simulink model "EngPrt_PrtLimMech1"  (R2016b)
settings: configuration reference "CodeGenConfigSet" (kept outside this file)
values from neighbouring files (symbols this model uses):
  EngPrt_facEngSPOffset_CUR = Calibration.Parameter    [init_EngPrt_PrtLimMech.m]    (also in init_EngPrt_PrtLimMech_SIL.m = Simulink.Parameter)
  EngPrt_facEngSPOffset_CURX = Calibration.Parameter    [init_EngPrt_PrtLimMech.m]    (also in init_EngPrt_PrtLimMech_SIL.m = Simulink.Parameter)
  EngPrt_facTrqLimCor_MAP = Calibration.Parameter    [init_EngPrt_PrtLimMech.m]    (also in init_EngPrt_PrtLimMech_SIL.m = Simulink.Parameter)
  EngPrt_facTrqLimCor_MAPX = Calibration.Parameter    [init_EngPrt_PrtLimMech.m]    (also in init_EngPrt_PrtLimMech_SIL.m = Simulink.Parameter)
  EngPrt_facTrqLimCor_MAPY = Calibration.Parameter    [init_EngPrt_PrtLimMech.m]    (also in init_EngPrt_PrtLimMech_SIL.m = Simulink.Parameter)
  EngPrt_nEngSplimOffset_C = Calibration.Parameter    [init_EngPrt_PrtLimMech.m]    (also in init_EngPrt_PrtLimMech_SIL.m = Simulink.Parameter)
  EngPrt_nEngSplimRmpSlopeNeg_C = Calibration.Parameter    [init_EngPrt_PrtLimMech.m]    (also in init_EngPrt_PrtLimMech_SIL.m = Simulink.Parameter)
  EngPrt_nEngSplimRmpSlopePos_C = Calibration.Parameter    [init_EngPrt_PrtLimMech.m]    (also in init_EngPrt_PrtLimMech_SIL.m = Simulink.Parameter)
  EngPrt_numTrqLim_C = Calibration.Parameter    [init_EngPrt_PrtLimMech.m]    (also in init_EngPrt_PrtLimMech_SIL.m = Simulink.Parameter)
  EngPrt_qLim_CUR = Calibration.Parameter    [init_EngPrt_PrtLimMech.m]    (also in init_EngPrt_PrtLimMech_SIL.m = Simulink.Parameter)
  EngPrt_qLim_CURX = Calibration.Parameter    [init_EngPrt_PrtLimMech.m]    (also in init_EngPrt_PrtLimMech_SIL.m = Simulink.Parameter)
  EngPrt_RmpLimNErrNeg_C = Calibration.Parameter    [init_EngPrt_PrtLimMech.m]    (also in init_EngPrt_PrtLimMech_SIL.m = Simulink.Parameter)
  EngPrt_RmpLimNErrPos_C = Calibration.Parameter    [init_EngPrt_PrtLimMech.m]    (also in init_EngPrt_PrtLimMech_SIL.m = Simulink.Parameter)
  EngPrt_swtLimCorType_C = Calibration.Parameter    [init_EngPrt_PrtLimMech.m]    (also in init_EngPrt_PrtLimMech_SIL.m = Simulink.Parameter)
  EngPrt_swtTrq_C = Calibration.Parameter    [init_EngPrt_PrtLimMech.m]    (also in init_EngPrt_PrtLimMech_SIL.m = Simulink.Parameter)
  EngPrt_trqLim_CUR = Calibration.Parameter    [init_EngPrt_PrtLimMech.m]    (also in init_EngPrt_PrtLimMech_SIL.m = Simulink.Parameter)
  EngPrt_trqLim_CURX = Calibration.Parameter    [init_EngPrt_PrtLimMech.m]    (also in init_EngPrt_PrtLimMech_SIL.m = Simulink.Parameter)
  EngPrt_trqLimAPSCor_MAP = Calibration.Parameter    [init_EngPrt_PrtLimMech.m]    (also in init_EngPrt_PrtLimMech_SIL.m = Simulink.Parameter)
  EngPrt_trqLimAPSCor_MAPX = Calibration.Parameter    [init_EngPrt_PrtLimMech.m]    (also in init_EngPrt_PrtLimMech_SIL.m = Simulink.Parameter)
  EngPrt_trqLimAPSCor_MAPY = Calibration.Parameter    [init_EngPrt_PrtLimMech.m]    (also in init_EngPrt_PrtLimMech_SIL.m = Simulink.Parameter)
  EngPrt_trqLimEngTempCor_MAP = Calibration.Parameter    [init_EngPrt_PrtLimMech.m]    (also in init_EngPrt_PrtLimMech_SIL.m = Simulink.Parameter)
  EngPrt_trqLimEngTempCor_MAPX = Calibration.Parameter    [init_EngPrt_PrtLimMech.m]    (also in init_EngPrt_PrtLimMech_SIL.m = Simulink.Parameter)
  EngPrt_trqLimEngTempCor_MAPY = Calibration.Parameter    [init_EngPrt_PrtLimMech.m]    (also in init_EngPrt_PrtLimMech_SIL.m = Simulink.Parameter)
  EngPrt_trqNLim_CUR = Calibration.Parameter    [init_EngPrt_PrtLimMech.m]    (also in init_EngPrt_PrtLimMech_SIL.m = Simulink.Parameter)
  EngPrt_trqNLim_CURX = Calibration.Parameter    [init_EngPrt_PrtLimMech.m]    (also in init_EngPrt_PrtLimMech_SIL.m = Simulink.Parameter)
  EngPrt_trqNLimSpr_CUR = Calibration.Parameter    [init_EngPrt_PrtLimMech.m]    (also in init_EngPrt_PrtLimMech_SIL.m = Simulink.Parameter)
  EngPrt_trqNLimSpr_CURX = Calibration.Parameter    [init_EngPrt_PrtLimMech.m]    (also in init_EngPrt_PrtLimMech_SIL.m = Simulink.Parameter)
undefined symbols (not defined in the file or in its folder): EngPrt_PrtLimMech_DT, Switch_conv
libraries: CXLib x8
settings Model: Creator=Administrator  LastModifiedBy=xuxingpei
settings ConfigSetRef: SourceLocation=Base Workspace

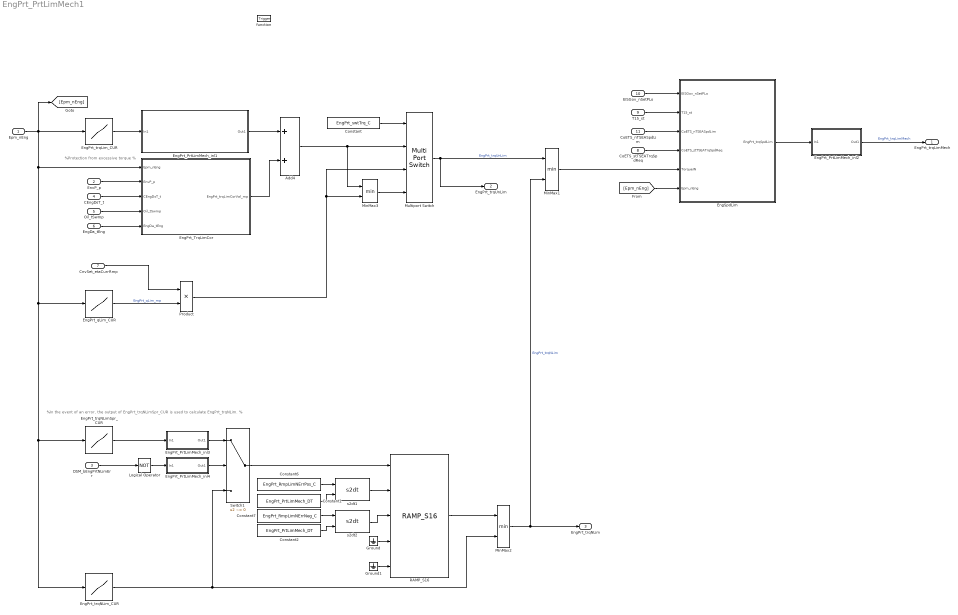
== system EngPrt_PrtLimMech1 ==
  note: %In the event of an error, the output of EngPrt_trqNLimSpr_CUR is used to calculate EngPrt_trqNLim. %
  note: %Protection from excessive torque %
  Epm_nEng : Inport  Tag=rpm  Description=Engine speed  OutMin=0  OutMax=6000  OutDataTypeStr=EngSpeed_rpm
  EnvP_p : Inport  Tag=kPa  Description=Barometric pressure  Port=2  OutMin=0  OutMax=3276  OutDataTypeStr=AirPressure_kPa
  DSM_bEngPrtNLimErr : Inport  Description=Activation of additional engine speed limitation  Port=3  OutMin=0  OutMax=1  OutDataTypeStr=boolean
  CEngDsT_t : Inport  Tag=deg  Description=engine coolant temperature after filter  Port=4  OutMin=-200  OutMax=200  OutDataTypeStr=Temp_deg
  Oil_tSwmp : Inport  Tag=deg  Description=Oil temperature in oil sump  Port=5  OutMin=-50  OutMax=200  OutDataTypeStr=Temp_deg
  EngDa_tEng : Inport  Tag=deg  Description=Engine temperature  Port=6  OutMin=-1000  OutMax=1000  OutDataTypeStr=Temp_deg
  CnvSet_etaCurrRmp : Inport  Tag=Nm/(mg/hub)  Description=Conversion efficiency corresponding to CnvSet_qSet  Port=7  OutMin=-255  OutMax=255  OutDataTypeStr=TrqEta_Nm_mg_hub
  CoETS_stTSEATrqSpdReq : Inport  Description=Status of information about torque and speed intervention  Port=8  OutMin=0  OutMax=65535  OutDataTypeStr=State_uint16
  T15_st : Inport  Description=Terminal 15 status after debouncing  Port=9  OutDataTypeStr=Enum: Switch_conv
  EISGov_nSetPLo : Inport  Tag=rpm  Description=Lower limit of the speed interval (set point speed) of the EISGov  Port=10  OutMin=0  OutMax=6000  OutDataTypeStr=EngSpeed_rpm
  CoETS_nTSEASpdLim : Inport  Tag=rpm  Description=|  Port=11  OutMin=0  OutMax=6000  OutDataTypeStr=EngSpeed_rpm
      | The engine speed limitation requested from TSC1
      | CAN messages. This engine speed limit is given to
      | the speed governor
  function : TriggerPort  TriggerType=function-call  VariantControl=Variant
  Add4 : Sum  InputSameDT=on
  Constant : Constant  Value=EngPrt_swtTrq_C
  Constant1 : Constant  Value=EngPrt_PrtLimMech_DT  OutDataTypeStr=Inherit: Inherit via back propagation
  Constant2 : Constant  Value=EngPrt_PrtLimMech_DT  OutDataTypeStr=Inherit: Inherit via back propagation
  Constant6 : Constant  Value=EngPrt_RmpLimNErrPos_C
  Constant7 : Constant  Value=EngPrt_RmpLimNErrNeg_C
  EngPrt_PrtLimMech_inl1 : Subsystem
  EngPrt_PrtLimMech_inl2 : Subsystem
  EngPrt_PrtLimMech_inl3 : Subsystem
  EngPrt_PrtLimMech_inl4 : Subsystem
  EngPrt_TrqLimCor : Subsystem
  EngPrt_qLim_CUR : Lookup_n-D  NumberOfTableDimensions=1  BreakpointsForDimension1=EngPrt_qLim_CURX  BreakpointsForDimension2=[1:3]  IndexSearchMethod=Linear search  Table=EngPrt_qLim_CUR  ExtrapMethod=Clip  InternalRulePriority=Speed  OutDataTypeStr=Inherit: Inherit via back propagation  RndMeth=Simplest  SaturateOnIntegerOverflow=on
  EngPrt_trqLim_CUR : Lookup_n-D  NumberOfTableDimensions=1  BreakpointsForDimension1=EngPrt_trqLim_CURX  BreakpointsForDimension2=[1:3]  IndexSearchMethod=Linear search  Table=EngPrt_trqLim_CUR  ExtrapMethod=Clip  InternalRulePriority=Speed  OutDataTypeStr=Inherit: Inherit via back propagation  RndMeth=Simplest  SaturateOnIntegerOverflow=on
  EngPrt_trqNLimSpr_CUR : Lookup_n-D  NumberOfTableDimensions=1  BreakpointsForDimension1=EngPrt_trqNLimSpr_CURX  BreakpointsForDimension2=[1:3]  IndexSearchMethod=Linear search  Table=EngPrt_trqNLimSpr_CUR  ExtrapMethod=Clip  InternalRulePriority=Speed  OutDataTypeStr=Inherit: Inherit via back propagation  RndMeth=Simplest  SaturateOnIntegerOverflow=on
  EngPrt_trqNLim_CUR : Lookup_n-D  NumberOfTableDimensions=1  BreakpointsForDimension1=EngPrt_trqNLim_CURX  BreakpointsForDimension2=[1:3]  IndexSearchMethod=Linear search  Table=EngPrt_trqNLim_CUR  ExtrapMethod=Clip  InternalRulePriority=Speed  OutDataTypeStr=Inherit: Inherit via back propagation  RndMeth=Simplest  SaturateOnIntegerOverflow=on
  EngSpdLim : Subsystem
  Ground : Ground
  Ground1 : Ground
  Logical Operator : Logic  Operator=NOT  AllPortsSameDT=off  OutDataTypeStr=boolean
  MinMax1 : MinMax  Inputs=2  InputSameDT=on
  MinMax2 : MinMax  Inputs=2  InputSameDT=on
  MinMax3 : MinMax  Inputs=2  InputSameDT=on
  Multiport Switch : MultiPortSwitch  DataPortOrder=Zero-based contiguous  OutDataTypeStr=Inherit: Inherit via back propagation  InputSameDT=on
  Product : Product  OutDataTypeStr=Inherit: Inherit via back propagation  SaturateOnIntegerOverflow=on
  RAMP_S16 : CXLib/RAMP_S16
  Switch1 : Switch  Criteria=u2 ~= 0  InputSameDT=on
  s2dt1 : CXLib/s2dt
  s2dt2 : CXLib/s2dt
  EngPrt_trqLimMech : Outport  Tag=Nm  Description=Resulting limiting torque for engine mechanics protection (inner engine torque)  OutMin=-3276.8  OutMax=3276.7  OutDataTypeStr=Trq_Nm
  EngPrt_trqUnLim : Outport  Tag=Nm  Description=Enabled torque from the maximum power manager  Port=2  OutMin=-3276.8  OutMax=3276.7  OutDataTypeStr=Trq_Nm
  EngPrt_trqNLim : Outport  Tag=Nm  Description=Limiting torque for protection from excessive engine speed  Port=3  OutMin=-3276.8  OutMax=3276.7  OutDataTypeStr=Trq_Nm
  wires:
  Epm_nEng/1 -> [Epm_nEng], EngPrt_qLim_CUR/1, EngPrt_trqNLim_CUR/1, EngPrt_trqNLimSpr_CUR/1, EngPrt_TrqLimCor/1(Epm_nEng), EngPrt_trqLim_CUR/1
  EngPrt_trqLim_CUR/1 -> EngPrt_PrtLimMech_inl1/1(In1)
  EngPrt_PrtLimMech_inl1/1(Out1) -> Add4/1
  EngPrt_TrqLimCor/1(EngPrt_trqLimCorVal_mp) -> Add4/2
  EngPrt_PrtLimMech_inl2/1(Out1) -> EngPrt_trqLimMech/1  "EngPrt_trqLimMech"
  MinMax2/1 -> MinMax1/2, EngPrt_trqNLim/1  "EngPrt_trqNLim"
  EngPrt_trqNLimSpr_CUR/1 -> EngPrt_PrtLimMech_inl3/1(In1)
  EngPrt_trqNLim_CUR/1 -> MinMax2/2, Switch1/3
  EnvP_p/1 -> EngPrt_TrqLimCor/2(EnvP_p)
  EngPrt_PrtLimMech_inl3/1(Out1) -> Switch1/1
  EngPrt_PrtLimMech_inl4/1(Out1) -> Switch1/2
  Ground/1 -> RAMP_S16/4
  Ground1/1 -> RAMP_S16/5
  DSM_bEngPrtNLimErr/1 -> Logical Operator/1
  Logical Operator/1 -> EngPrt_PrtLimMech_inl4/1(In1)
  Constant7/1 -> s2dt2/1
  Switch1/1 -> RAMP_S16/1
  RAMP_S16/1 -> MinMax2/1
  Constant6/1 -> s2dt1/1
  s2dt1/1 -> RAMP_S16/2
  Constant1/1 -> s2dt1/2
  s2dt2/1 -> RAMP_S16/3
  Constant2/1 -> s2dt2/2
  Oil_tSwmp/1 -> EngPrt_TrqLimCor/4(Oil_tSwmp)
  EngDa_tEng/1 -> EngPrt_TrqLimCor/5(EngDa_tEng)
  CEngDsT_t/1 -> EngPrt_TrqLimCor/3(CEngDsT_t)
  Multiport Switch/1 -> EngPrt_trqUnLim/1, MinMax1/1  "EngPrt_trqUnLim"
  EngPrt_qLim_CUR/1 -> Product/2  "EngPrt_qLim_mp"
  CnvSet_etaCurrRmp/1 -> Product/1
  Add4/1 -> Multiport Switch/2, MinMax3/1
  Product/1 -> Multiport Switch/3, MinMax3/2
  MinMax3/1 -> Multiport Switch/4
  Constant/1 -> Multiport Switch/1
  EISGov_nSetPLo/1 -> EngSpdLim/1(EISGov_nSetPLo)
  T15_st/1 -> EngSpdLim/2(T15_st)
  CoETS_nTSEASpdLim/1 -> EngSpdLim/3(CoETS_nTSEASpdLim)
  CoETS_stTSEATrqSpdReq/1 -> EngSpdLim/4(CoETS_stTSEATrqSpdReq)
  EngSpdLim/1(EngPrt_trqSpdLim) -> EngPrt_PrtLimMech_inl2/1(In1)
  MinMax1/1 -> EngSpdLim/5(TorqueIN)
  [Epm_nEng] -> EngSpdLim/6(Epm_nEng)

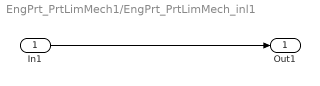
== system EngPrt_PrtLimMech1/EngPrt_PrtLimMech_inl1 ==
  In1 : Inport
  Out1 : Outport
  wires:
  In1/1 -> Out1/1

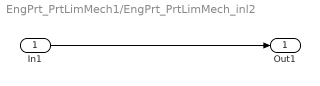
== system EngPrt_PrtLimMech1/EngPrt_PrtLimMech_inl2 ==
  In1 : Inport
  Out1 : Outport
  wires:
  In1/1 -> Out1/1

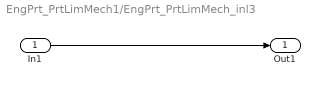
== system EngPrt_PrtLimMech1/EngPrt_PrtLimMech_inl3 ==
  In1 : Inport
  Out1 : Outport
  wires:
  In1/1 -> Out1/1

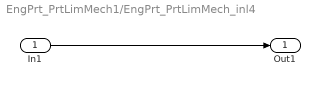
== system EngPrt_PrtLimMech1/EngPrt_PrtLimMech_inl4 ==
  In1 : Inport
  Out1 : Outport
  wires:
  In1/1 -> Out1/1

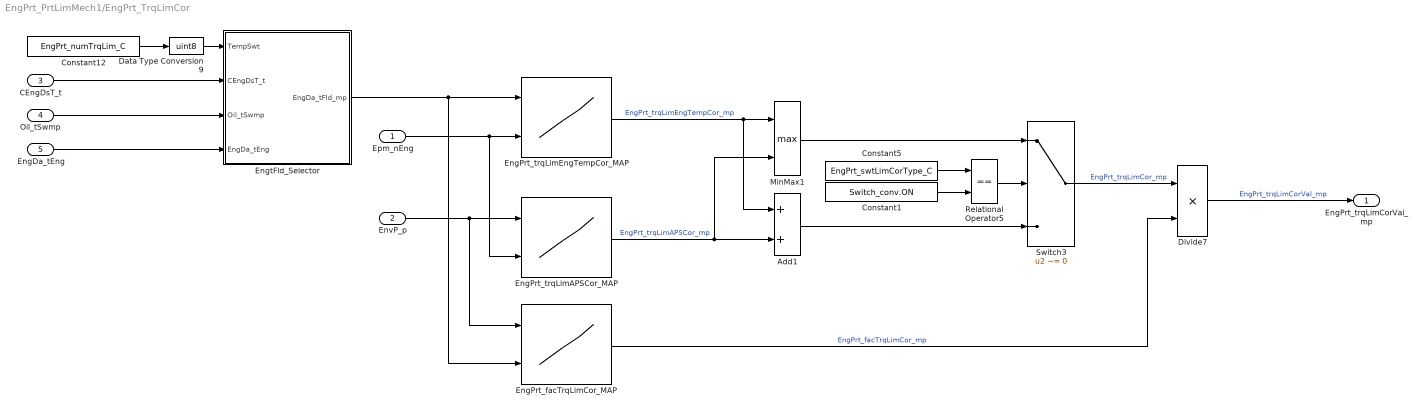
== system EngPrt_PrtLimMech1/EngPrt_TrqLimCor ==
  Epm_nEng : Inport
  EnvP_p : Inport  Port=2
  CEngDsT_t : Inport  Tag=deg  Description=engine coolant temperature after filter  Port=3  OutMin=-200  OutMax=200  OutDataTypeStr=Temp_deg
  Oil_tSwmp : Inport  Tag=deg  Description=Oil temperature in oil sump  Port=4  OutMin=-50  OutMax=200  OutDataTypeStr=Temp_deg
  EngDa_tEng : Inport  Tag=deg  Description=Engine temperature  Port=5  OutMin=-1000  OutMax=1000  OutDataTypeStr=Temp_deg
  Add1 : Sum  InputSameDT=on
  Constant1 : Constant  Value=Switch_conv.ON  OutDataTypeStr=Inherit: Inherit via back propagation
  Constant12 : Constant  Value=EngPrt_numTrqLim_C  SampleTime=-1
  Constant5 : Constant  Value=EngPrt_swtLimCorType_C
  Data Type Conversion9 : DataTypeConversion  OutDataTypeStr=uint8
  Divide7 : Product  Inputs=**  OutDataTypeStr=Trq_Nm
  EngPrt_facTrqLimCor_MAP : Lookup_n-D  DialogController=Simulink.DDGSource  BreakpointsForDimension1=EngPrt_facTrqLimCor_MAPY  BreakpointsForDimension2=EngPrt_facTrqLimCor_MAPX  IndexSearchMethod=Linear search  BeginIndexSearchUsingPreviousIndexResult=on  Table=EngPrt_facTrqLimCor_MAP  ExtrapMethod=Clip  UseLastTableValue=on  InternalRulePriority=Speed  OutDataTypeStr=Inherit: Inherit via back propagation  SaturateOnIntegerOverflow=on
  EngPrt_trqLimAPSCor_MAP : Lookup_n-D  DialogController=Simulink.DDGSource  BreakpointsForDimension1=EngPrt_trqLimAPSCor_MAPY  BreakpointsForDimension2=EngPrt_trqLimAPSCor_MAPX  IndexSearchMethod=Linear search  BeginIndexSearchUsingPreviousIndexResult=on  Table=EngPrt_trqLimAPSCor_MAP  ExtrapMethod=Clip  UseLastTableValue=on  InternalRulePriority=Speed  OutDataTypeStr=Inherit: Inherit via back propagation  SaturateOnIntegerOverflow=on
  EngPrt_trqLimEngTempCor_MAP : Lookup_n-D  DialogController=Simulink.DDGSource  BreakpointsForDimension1=EngPrt_trqLimEngTempCor_MAPY  BreakpointsForDimension2=EngPrt_trqLimEngTempCor_MAPX  IndexSearchMethod=Linear search  BeginIndexSearchUsingPreviousIndexResult=on  Table=EngPrt_trqLimEngTempCor_MAP  ExtrapMethod=Clip  UseLastTableValue=on  InternalRulePriority=Speed  OutDataTypeStr=Inherit: Inherit via back propagation  SaturateOnIntegerOverflow=on
  EngtFld_Selector : Subsystem
  MinMax1 : MinMax  Function=max  Inputs=2  InputSameDT=on
  Relational Operator5 : RelationalOperator  Operator===  OutDataTypeStr=boolean  RndMeth=Simplest  InputSameDT=on
  Switch3 : Switch  Criteria=u2 ~= 0  InputSameDT=on
  EngPrt_trqLimCorVal_mp : Outport
  wires:
  Constant1/1 -> Relational Operator5/2
  Relational Operator5/1 -> Switch3/2
  Epm_nEng/1 -> EngPrt_trqLimAPSCor_MAP/2, EngPrt_trqLimEngTempCor_MAP/2
  EngtFld_Selector/1(EngDa_tFld_mp) -> EngPrt_facTrqLimCor_MAP/2, EngPrt_trqLimEngTempCor_MAP/1
  EnvP_p/1 -> EngPrt_facTrqLimCor_MAP/1, EngPrt_trqLimAPSCor_MAP/1
  EngPrt_facTrqLimCor_MAP/1 -> Divide7/2  "EngPrt_facTrqLimCor_mp"
  EngPrt_trqLimAPSCor_MAP/1 -> MinMax1/2, Add1/2  "EngPrt_trqLimAPSCor_mp"
  EngPrt_trqLimEngTempCor_MAP/1 -> Add1/1, MinMax1/1  "EngPrt_trqLimEngTempCor_mp"
  Add1/1 -> Switch3/3
  MinMax1/1 -> Switch3/1
  Constant5/1 -> Relational Operator5/1
  Divide7/1 -> EngPrt_trqLimCorVal_mp/1  "EngPrt_trqLimCorVal_mp"
  Switch3/1 -> Divide7/1  "EngPrt_trqLimCor_mp"
  Constant12/1 -> Data Type Conversion9/1
  Data Type Conversion9/1 -> EngtFld_Selector/1(TempSwt)
  CEngDsT_t/1 -> EngtFld_Selector/2(CEngDsT_t)
  Oil_tSwmp/1 -> EngtFld_Selector/3(Oil_tSwmp)
  EngDa_tEng/1 -> EngtFld_Selector/4(EngDa_tEng)

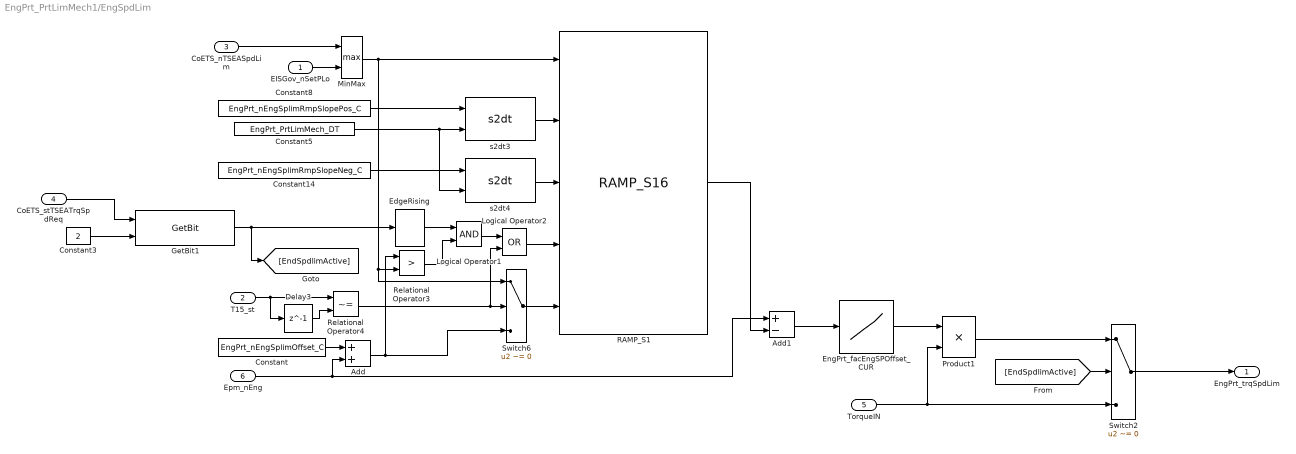
== system EngPrt_PrtLimMech1/EngSpdLim ==
  EISGov_nSetPLo : Inport  Tag=rpm  Description=Lower limit of the speed interval (set point speed) of the EISGov  OutMin=0  OutMax=6000  OutDataTypeStr=EngSpeed_rpm
  T15_st : Inport  Description=Terminal 15 status after debouncing  Port=2  OutDataTypeStr=Enum: Switch_conv
  CoETS_nTSEASpdLim : Inport  Tag=rpm  Description=The engine speed limitation requested from TSC1 CAN messages. This engine speed limit is given to the speed governor.  Port=3  OutMin=-16384  OutMax=16383.5  OutDataTypeStr=EngSpeed_rpm
  CoETS_stTSEATrqSpdReq : Inport  Description=Status of information about torque and speed intervention  Port=4  OutMin=0  OutMax=65535  OutDataTypeStr=State_uint16
  TorqueIN : Inport  Port=5
  Epm_nEng : Inport  Tag=rpm  Description=Engine speed  Port=6  OutMin=0  OutMax=6000  OutDataTypeStr=EngSpeed_rpm
  Add : Sum
  Add1 : Sum  Inputs=+-  SaturateOnIntegerOverflow=on
  Constant : Constant  Value=EngPrt_nEngSplimOffset_C
  Constant14 : Constant  Value=EngPrt_nEngSplimRmpSlopeNeg_C
  Constant3 : Constant  Value=2  OutDataTypeStr=Inherit: Inherit via back propagation
  Constant5 : Constant  Value=EngPrt_PrtLimMech_DT
  Constant8 : Constant  Value=EngPrt_nEngSplimRmpSlopePos_C
  Delay3 : Delay  DelayLength=1  InitialCondition=Switch_conv.OFF
  EdgeRising : CXLib/EdgeRising
  EngPrt_facEngSPOffset_CUR : Lookup_n-D  NumberOfTableDimensions=1  BreakpointsForDimension1=EngPrt_facEngSPOffset_CURX  BreakpointsForDimension2=[1:3]  IndexSearchMethod=Linear search  Table=EngPrt_facEngSPOffset_CUR  ExtrapMethod=Clip  InternalRulePriority=Speed  OutDataTypeStr=Inherit: Inherit via back propagation  RndMeth=Simplest  SaturateOnIntegerOverflow=on
  GetBit1 : CXLib/GetBit  dataTypeString=uint16  dataLength=0
      settings: AttributesFormatString=Get bit from %<dataTypeString>
  Logical Operator1 : Logic  AllPortsSameDT=off  OutDataTypeStr=boolean
  Logical Operator2 : Logic  Operator=OR  AllPortsSameDT=off  OutDataTypeStr=boolean
  MinMax : MinMax  Function=max  Inputs=2
  Product1 : Product  OutDataTypeStr=Inherit: Inherit via back propagation  SaturateOnIntegerOverflow=on
  RAMP_S1 : CXLib/RAMP_S16
  Relational Operator3 : RelationalOperator  Operator=>  OutDataTypeStr=boolean  RndMeth=Simplest
  Relational Operator4 : RelationalOperator  Operator=~=  OutDataTypeStr=boolean  RndMeth=Simplest
  Switch2 : Switch  Criteria=u2 ~= 0  InputSameDT=on
  Switch6 : Switch  Criteria=u2 ~= 0
  s2dt3 : CXLib/s2dt
  s2dt4 : CXLib/s2dt
  EngPrt_trqSpdLim : Outport  Tag=Nm  Description=Enabled torque from the maximum power manager  OutMin=-3276.8  OutMax=3276.7  OutDataTypeStr=Trq_Nm
  wires:
  Switch2/1 -> EngPrt_trqSpdLim/1
  Product1/1 -> Switch2/1
  EngPrt_facEngSPOffset_CUR/1 -> Product1/1
  Epm_nEng/1 -> Add1/1, Add/2
  CoETS_nTSEASpdLim/1 -> MinMax/1
  TorqueIN/1 -> Product1/2, Switch2/3
  GetBit1/1 -> [EndSpdlimActive], EdgeRising/1
  EdgeRising/1 -> Logical Operator1/1
  Relational Operator3/1 -> Logical Operator1/2
  RAMP_S1/1 -> Add1/2
  T15_st/1 -> Relational Operator4/1, Delay3/1
  s2dt4/1 -> RAMP_S1/3
  EISGov_nSetPLo/1 -> MinMax/2
  Logical Operator1/1 -> Logical Operator2/1
  Add1/1 -> EngPrt_facEngSPOffset_CUR/1
  Constant5/1 -> s2dt4/2, s2dt3/2
  Delay3/1 -> Relational Operator4/2
  Logical Operator2/1 -> RAMP_S1/4
  Relational Operator4/1 -> Logical Operator2/2, Switch6/2
  Switch6/1 -> RAMP_S1/5
  s2dt3/1 -> RAMP_S1/2
  MinMax/1 -> Switch6/1, Relational Operator3/2, RAMP_S1/1
  Constant8/1 -> s2dt3/1
  Constant14/1 -> s2dt4/1
  Constant3/1 -> GetBit1/2
  CoETS_stTSEATrqSpdReq/1 -> GetBit1/1
  [EndSpdlimActive] -> Switch2/2
  Add/1 -> Switch6/3, Relational Operator3/1
  Constant/1 -> Add/1

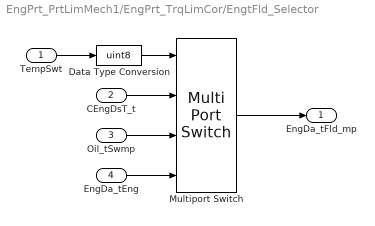
== system EngPrt_PrtLimMech1/EngPrt_TrqLimCor/EngtFld_Selector ==
  TempSwt : Inport
  CEngDsT_t : Inport  Tag=deg  Description=engine coolant temperature after filter  Port=2
  Oil_tSwmp : Inport  Tag=deg  Description=Oil temperature in oil sump  Port=3
  EngDa_tEng : Inport  Tag=deg  Description=Engine temperature  Port=4
  Data Type Conversion : DataTypeConversion  OutDataTypeStr=uint8
  Multiport Switch : MultiPortSwitch  DataPortOrder=Zero-based contiguous
  EngDa_tFld_mp : Outport  Tag=deg  Description=Engine temperature field
  wires:
  CEngDsT_t/1 -> Multiport Switch/2
  Multiport Switch/1 -> EngDa_tFld_mp/1
  EngDa_tEng/1 -> Multiport Switch/4
  Oil_tSwmp/1 -> Multiport Switch/3
  Data Type Conversion/1 -> Multiport Switch/1
  TempSwt/1 -> Data Type Conversion/1
